simulink model "run_sim_paper_scenario"  (R2020a)
settings: Solver=ode4  StartTime=0.0  StopTime=30.0  FixedStep=0.01  RelTol=1e-3
values from neighbouring files (symbols this model uses):
  alfa_theta = 20    [init_sim_paper_scenario.m]
  alfa_theta_obs = 100    [init_sim_paper_scenario.m]
  beta1 = 1.2    [init_sim_paper_scenario.m]
  beta2 = 0.8    [init_sim_paper_scenario.m]
  beta_Phi_1 = pp0 * cal_frac_squ( 3, p_p0_plus_1, q_p0_plus_1 )                          * cal_frac_squ( eps_s_bar / pi, p_p0_min_2, q_p0_min_2 )                          / ( 2 * ( 2 * pp0 - 1 ) * tanh( gamma0 * ( eps_s_bar / pi ) / 2 ) )                          - ( cal_frac_squ( 3, p_p0_plus_1, q_p0_plus_1 ) * gamma0 / ( 4 * ( 2 * pp0 -1 ) ) )                          * cal_frac_squ( eps_s_bar / pi, p_p0_min_ ...(+136 chars)    [init_sim_paper_scenario.m]
  beta_Phi_2 = ( 1 - pp0 ) * cal_frac_squ( 3, p_p0_plus_1, q_p0_plus_1 )                          / ( 2 * ( 1 - 2 * pp0 ) * cal_frac_squ( eps_s_bar / pi, p_p0_0, q_p0_0 ) * tanh( gamma0 * ( eps_s_bar / pi ) / 2 ) )                          - ( cal_frac_squ( 3, p_p0_plus_1, q_p0_plus_1 ) * gamma0 / ( 4 * ( 1 - 2 * pp0 ) ) )                          * cal_frac_squ( eps_s_bar / pi, p_1_min_p0, q_1_min_p0 )          ...(+112 chars)    [init_sim_paper_scenario.m]
  c1_diff_sigma_bar_v = diag([25; 30; 20])    [init_sim_paper_scenario.m]
  c1_diff_sigma_bar_w = diag([12; 12; 12])    [init_sim_paper_scenario.m]
  c1_diff_ui = diag([25; 30; 20])    [init_sim_paper_scenario.m]
  c1v = diag([5.8; 6.5; 6.5])    [init_sim_paper_scenario.m]
  c2_diff_sigma_bar_v = diag([50; 50; 10])    [init_sim_paper_scenario.m]
  c2_diff_sigma_bar_w = diag([12; 12; 12])    [init_sim_paper_scenario.m]
  c2_diff_ui = diag([50; 50; 10])    [init_sim_paper_scenario.m]
  c2v = diag([5.8; 6.5; 6.5])    [init_sim_paper_scenario.m]
  c3_diff_sigma_bar_v = diag([15; 15; 10])    [init_sim_paper_scenario.m]
  c3_diff_sigma_bar_w = diag([15; 15; 15])    [init_sim_paper_scenario.m]
  c3_diff_ui = diag([15; 15; 10])    [init_sim_paper_scenario.m]
  c3v = diag([4.8; 6.4; 6.0])    [init_sim_paper_scenario.m]
  c_w_1 = diag( [20; 15; 15] )    [init_sim_paper_scenario.m]
  c_w_2 = diag( [20; 15; 15] )    [init_sim_paper_scenario.m]
  c_w_3 = diag( [2; 2; 2] )    [init_sim_paper_scenario.m]
  cS0 = diag( [4.5; 4.5; 4.5] )    [init_sim_paper_scenario.m]
  delta_p_i_0 = zeros(3, NF)    [init_sim_paper_scenario.m]
  delta_v_i_0 = zeros(3, NF)    [init_sim_paper_scenario.m]
  dp_aa_t = 0.2 * ones(3, 5) + ( 1.0 - 0.2 ) * rand(3, 5)    [init_sim_paper_scenario.m]
  dp_ff_t = [ 0.4 * ones(1, 5) + ( 1.0 - 0.4 ) * rand(1, 5);                      0.4 * ones(1, 5) + ( 1.0 - 0.4 ) * rand(1, 5);                      0.2 * ones(1, 5) + ( 0.6 - 0.2 ) * rand(1, 5) ]    [init_sim_paper_scenario.m]
  dp_phi_t = ( - pi / 2 ) * ones(3, 5) + ( pi / 2 - ( - pi / 2 ) ) * rand(3, 5)    [init_sim_paper_scenario.m]
  dw_aa_t = 0.2 * ones(3, 5) + ( 1.0 - 0.2 ) * rand(3, 5)    [init_sim_paper_scenario.m]
  dw_ff_t = [ 0.4 * ones(1, 5) + ( 1.0 - 0.4 ) * rand(1, 5);                      0.4 * ones(1, 5) + ( 1.0 - 0.4 ) * rand(1, 5);                      0.2 * ones(1, 5) + ( 0.6 - 0.2 ) * rand(1, 5) ]    [init_sim_paper_scenario.m]
  dw_phi_t = ( - pi / 2 ) * ones(3, 5) + ( pi / 2 - ( - pi / 2 ) ) * rand(3, 5)    [init_sim_paper_scenario.m]
  dwci_init = zeros(3,5)    [init_sim_paper_scenario.m]
  eps_s_bar_div_pi = eps_s_bar / pi    (= 0.03)    [init_sim_paper_scenario.m]
  etai_0 = zeros(3,5)    [init_sim_paper_scenario.m]
  gamma0 = 20    [init_sim_paper_scenario.m]
  h1w = diag([20.0; 20.0; 20.0])    [init_sim_paper_scenario.m]
  h2w = diag([30.0; 35.0; 35.0])    [init_sim_paper_scenario.m]
  h3w = diag([30.0; 25.0; 30.0])    [init_sim_paper_scenario.m]
  Ji = zeros(3,3,NF)    [init_sim_paper_scenario.m]
  k_J_0 = diag( [1; 1; 1] )    [init_sim_paper_scenario.m]
  kai_1_t = 0.02    [init_sim_paper_scenario.m]
  kai_3_t = 0.1    [init_sim_paper_scenario.m]
  kai_chi_1 = diag([6; 6; 6])    [init_sim_paper_scenario.m]
  kai_chi_2 = diag([6; 6; 6])    [init_sim_paper_scenario.m]
  kai_u_1 = diag([8; 8; 8])    [init_sim_paper_scenario.m]
  kai_u_2 = diag([8; 8; 8])    [init_sim_paper_scenario.m]
  ksii_0 = zeros(3,5)    [init_sim_paper_scenario.m]
  l1v = diag([20; 20; 20])    [init_sim_paper_scenario.m]
  l2v = diag([30; 30; 30])    [init_sim_paper_scenario.m]
  Lamd_diff_sigma_bar_v = 0.5    [init_sim_paper_scenario.m]
  Lamd_diff_sigma_bar_w = 0.8    [init_sim_paper_scenario.m]
  Lamd_diff_ui = 0.8    [init_sim_paper_scenario.m]
  mass_i = zeros(1,NF)    [init_sim_paper_scenario.m]
  Mii = diag([1;0;0;0;1])    [init_sim_paper_scenario.m]
  mu_c_theta = 100    [init_sim_paper_scenario.m]
  mu_d_w = 100    [init_sim_paper_scenario.m]
  pos0 = zeros(3, 1)    [init_sim_paper_scenario.m]
  pp0 = 8 / 11    (= 0.727272727273)    [init_sim_paper_scenario.m]    (also in plot_sim_paper_scenario.m = plot3( ksi0(1, kkt), ksi0(2, kkt), ksi0(3, kkt),            )
  PZ0 = P0(3)    [init_sim_paper_scenario.m]
  PZ1 = 10    [init_sim_paper_scenario.m]
  Qci_init = repmat([1;0;0;0],1,NF)    [init_sim_paper_scenario.m]
  R0 = 4    [init_sim_paper_scenario.m]
  R1 = 8    [init_sim_paper_scenario.m]
  Rci_init = zeros(3,3,NF)    [init_sim_paper_scenario.m]
  Ri_init = zeros(3,3,NF)    [init_sim_paper_scenario.m]
  Rx2 = 10    [init_sim_paper_scenario.m]
  Ry2 = 6    [init_sim_paper_scenario.m]
  Rz2 = 4    [init_sim_paper_scenario.m]
  T0 = 0    [init_sim_paper_scenario.m]
  T1 = tseq1    (= 10)    [init_sim_paper_scenario.m]
  T12 = tseq1 + tseq12    (= 20)    [init_sim_paper_scenario.m]
  T2 = tseq1 + tseq12 + tseq2    (= 30)    [init_sim_paper_scenario.m]
  theta0 = ( 2 / 5 ) * pi    (= 1.25663706144)    [init_sim_paper_scenario.m]
  thr_p_plus_1 = cal_frac_squ( 3, p_p0_plus_1, q_p0_plus_1 )    [init_sim_paper_scenario.m]
  ui_init = zeros(3,NF)    [init_sim_paper_scenario.m]
  vel0 = zeros(3, 1)    [init_sim_paper_scenario.m]
  wci_init = zeros(3,5)    [init_sim_paper_scenario.m]
  Wij = [0,0,1,0,0;              0,0,1,1,0;              1,0,0,0,1;              0,1,1,0,0;              0,0,1,0,0]    [init_sim_paper_scenario.m]
  X1 = 8    [init_sim_paper_scenario.m]
  X2 = 2    [init_sim_paper_scenario.m]
  X3 = 3    [init_sim_paper_scenario.m]
  Y1 = 10    [init_sim_paper_scenario.m]
  Y2 = 2    [init_sim_paper_scenario.m]
  Y3 = 4    [init_sim_paper_scenario.m]
  Z1 = 4    [init_sim_paper_scenario.m]
  Z2 = -6    [init_sim_paper_scenario.m]
  Z3 = 2    [init_sim_paper_scenario.m]
  zeta_diff_sigma_bar_v = 0.08    [init_sim_paper_scenario.m]
  zeta_diff_sigma_bar_w = 0.3    [init_sim_paper_scenario.m]
  zeta_diff_ui = 0.05    [init_sim_paper_scenario.m]
undefined symbols (not defined in the file or in its folder): cal_frac_squ, p_2_p0, p_alfav1, p_alfav2, p_alfaw1, p_alfaw2, p_beta1, p_beta2, p_beta_w_1, p_beta_w_2, p_dbeta1, p_dbeta2, p_gamma1_pos, p_gamma1_vel, p_gamma2_pos, p_gamma2_vel, p_p0_min_1, p_p0_plus_1, q_2_p0, q_alfav1, q_alfav2, q_alfaw1, q_alfaw2, q_beta1, q_beta2, q_beta_w_1, q_beta_w_2, q_dbeta1, q_dbeta2, q_gamma1_pos, q_gamma1_vel, q_gamma2_pos, q_gamma2_vel, q_p0_min_1, q_p0_plus_1, Qei_init, Qi_init, Rei_init, V_Phi_Rei_init, wei_init, wi_init
(part 8 of 10)

== matlab function run_sim_paper_scenario/cal abs 72 ==
  data: x input; y output
function y = fcn(x)
y = abs(x(:));

== matlab function run_sim_paper_scenario/cal abs 73 ==
  data: x input; y output
function y = fcn(x)
y = abs(x(:));

== matlab function run_sim_paper_scenario/cal abs 74 ==
  data: x input; y output
function y = fcn(x)
y = abs(x(:));

== matlab function run_sim_paper_scenario/cal abs 75 ==
  data: x input; y output
function y = fcn(x)
y = abs(x(:));

== matlab function run_sim_paper_scenario/cal abs 76 ==
  data: x input; y output
function y = fcn(x)
y = abs(x(:));

== matlab function run_sim_paper_scenario/cal abs 77 ==
  data: x input; y output
function y = fcn(x)
y = abs(x(:));

== matlab function run_sim_paper_scenario/cal abs 78 ==
  data: x input; y output
function y = fcn(x)
y = abs(x(:));

== matlab function run_sim_paper_scenario/cal abs 79 ==
  data: x input; y output
function y = fcn(x)
y = abs(x(:));

== matlab function run_sim_paper_scenario/cal abs 80 ==
  data: x input; y output
function y = fcn(x)
y = abs(x(:));

== matlab function run_sim_paper_scenario/cal abs 81 ==
  data: x input; y output
function y = fcn(x)
y = abs(x(:));

== matlab function run_sim_paper_scenario/trans to column6 ==
  data: x input; y output
function y = fcn(x)
y = x(:);

== matlab function run_sim_paper_scenario/cal abs 82 ==
  data: x input; y output
function y = fcn(x)
y = abs(x(:));

== matlab function run_sim_paper_scenario/cal abs 83 ==
  data: x input; y output
function y = fcn(x)
y = abs(x(:));

== matlab function run_sim_paper_scenario/cal abs 84 ==
  data: x input; y output
function y = fcn(x)
y = abs(x(:));

== matlab function run_sim_paper_scenario/cal abs 85 ==
  data: x input; y output
function y = fcn(x)
y = abs(x(:));

== matlab function run_sim_paper_scenario/cal abs 86 ==
  data: x input; y output
function y = fcn(x)
y = abs(x(:));

== matlab function run_sim_paper_scenario/cal abs 87 ==
  data: x input; y output
function y = fcn(x)
y = abs(x(:));

== matlab function run_sim_paper_scenario/cal abs 88 ==
  data: x input; y output
function y = fcn(x)
y = abs(x(:));

== matlab function run_sim_paper_scenario/cal abs 89 ==
  data: x input; y output
function y = fcn(x)
y = abs(x(:));

== matlab function run_sim_paper_scenario/cal abs 90 ==
  data: x input; y output
function y = fcn(x)
y = abs(x(:));

== matlab function run_sim_paper_scenario/cal abs 91 ==
  data: x input; y output
function y = fcn(x)
y = abs(x(:));

== matlab function run_sim_paper_scenario/trans to column7 ==
  data: x input; y output
function y = fcn(x)
y = x(:);

== matlab function run_sim_paper_scenario/cal abs 92 ==
  data: x input; y output
function y = fcn(x)
y = abs(x(:));

== matlab function run_sim_paper_scenario/cal abs 93 ==
  data: x input; y output
function y = fcn(x)
y = abs(x(:));

== matlab function run_sim_paper_scenario/cal abs 94 ==
  data: x input; y output
function y = fcn(x)
y = abs(x(:));

== matlab function run_sim_paper_scenario/cal abs 95 ==
  data: x input; y output
function y = fcn(x)
y = abs(x(:));

== matlab function run_sim_paper_scenario/cal combine sigma_bar_w_tilt ==
  data: sigma_bar_w_vec input; sigma_bar_w_hat_vec input; sigma_bar_w_tilt_vec output
function sigma_bar_w_tilt_vec = fcn(sigma_bar_w_vec, sigma_bar_w_hat_vec)
%%%% observation error of virtual angular velocity control variable
sigma_bar_w_tilt_vec = zeros(3,5);
for iiuav = 1:5
    sigma_bar_w_tilt_vec(:,iiuav) = sigma_bar_w_vec(:,iiuav) - sigma_bar_w_hat_vec(:,iiuav);
end

== matlab function run_sim_paper_scenario/cal d_sigma_w agent 1 ==
  data: h3w input; d_sigma_w_1 output; Ji input; wi_vec input; taui_vec input; sigma_w_bar_vec input
function d_sigma_w_1 = fcn(h3w, Ji, wi_vec, taui_vec, sigma_w_bar_vec)
%%%% auxiliary angular velocity derivative
iiuav = 1;
d_sigma_w_1 = inv(Ji(:,:,iiuav)) * ( -cal_askew_mat(wi_vec(:,iiuav)) * Ji(:,:,iiuav) * wi_vec(:,iiuav) ...
                            + taui_vec(:,iiuav) + h3w * sigma_w_bar_vec(:,iiuav) );

== matlab function run_sim_paper_scenario/cal d_sigma_w agent 2 ==
  data: h3w input; d_sigma_w_2 output; Ji input; wi_vec input; taui_vec input; sigma_w_bar_vec input
function d_sigma_w_2 = fcn(h3w, Ji, wi_vec, taui_vec, sigma_w_bar_vec)
%%%% auxiliary angular velocity derivative
iiuav = 2;
d_sigma_w_2 = inv(Ji(:,:,iiuav)) * ( -cal_askew_mat(wi_vec(:,iiuav)) * Ji(:,:,iiuav) * wi_vec(:,iiuav) ...
                            + taui_vec(:,iiuav) + h3w * sigma_w_bar_vec(:,iiuav) );

== matlab function run_sim_paper_scenario/cal d_sigma_w agent 3 ==
  data: h3w input; d_sigma_w_3 output; Ji input; wi_vec input; taui_vec input; sigma_w_bar_vec input
function d_sigma_w_3 = fcn(h3w, Ji, wi_vec, taui_vec, sigma_w_bar_vec)
%%%% auxiliary angular velocity derivative
iiuav = 3;
d_sigma_w_3 = inv(Ji(:,:,iiuav)) * ( -cal_askew_mat(wi_vec(:,iiuav)) * Ji(:,:,iiuav) * wi_vec(:,iiuav) ...
                            + taui_vec(:,iiuav) + h3w * sigma_w_bar_vec(:,iiuav) );

== matlab function run_sim_paper_scenario/uav translational dynamics agent 1 ==
  data: dvi output; Ri input; ui input; dp input
function dvi = fcn(Ri, ui, dp)
%%%% update translational velocity dynamics
iiuav = 1;
g0 = 9.80663;
e3 = [0;0;1];
dvi = -g0 * e3 + norm(ui(:,iiuav),2) * Ri(:,:,iiuav) * e3 + dp(:,iiuav);

== matlab function run_sim_paper_scenario/cal d_sigma_w agent 4 ==
  data: h3w input; d_sigma_w_4 output; Ji input; wi_vec input; taui_vec input; sigma_w_bar_vec input
function d_sigma_w_4 = fcn(h3w, Ji, wi_vec, taui_vec, sigma_w_bar_vec)
%%%% auxiliary angular velocity derivative
iiuav = 4;
d_sigma_w_4 = inv(Ji(:,:,iiuav)) * ( -cal_askew_mat(wi_vec(:,iiuav)) * Ji(:,:,iiuav) * wi_vec(:,iiuav) ...
                            + taui_vec(:,iiuav) + h3w * sigma_w_bar_vec(:,iiuav) );

== matlab function run_sim_paper_scenario/cal d_sigma_w agent 5 ==
  data: h3w input; d_sigma_w_5 output; Ji input; wi_vec input; taui_vec input; sigma_w_bar_vec input
function d_sigma_w_5 = fcn(h3w, Ji, wi_vec, taui_vec, sigma_w_bar_vec)
%%%% auxiliary angular velocity derivative
iiuav = 5;
d_sigma_w_5 = inv(Ji(:,:,iiuav)) * ( -cal_askew_mat(wi_vec(:,iiuav)) * Ji(:,:,iiuav) * wi_vec(:,iiuav) ...
                            + taui_vec(:,iiuav) + h3w * sigma_w_bar_vec(:,iiuav) );

== matlab function run_sim_paper_scenario/cal duihat d2uihat by high-order differentiator node 1 ==
  data: c1 input; d_ui_hat output; d_dui_hat output; d_d2ui_hat output; c2 input; c3 input; chi_t input; ui_sig_1 input; ui_sig_2 input; ui_sig_3 input; ui_sig_4 input; ui_sig_5 input; ui_sig_6 input; dui_hat input; d2ui_hat input
function [d_ui_hat, d_dui_hat, d_d2ui_hat] = fcn(c1, c2, c3, chi_t, ui_sig_1, ui_sig_2, ui_sig_3, ...
                                                                                        ui_sig_4, ui_sig_5, ui_sig_6, dui_hat, d2ui_hat)
%%%% high-order sliding mode differentiator
d_d2ui_hat = -chi_t .* c1 * ui_sig_1(:) - (1 - chi_t) .* c1 * ui_sig_2(:);
d_dui_hat = -chi_t .* c2 * ui_sig_3(:) - (1 - chi_t) .* c2 * ui_sig_4(:) + d2ui_hat(:);
d_ui_hat = -chi_t .* c3 * ui_sig_5(:) - (1 - chi_t) .* c3 * ui_sig_6(:) + dui_hat(:);

== matlab function run_sim_paper_scenario/cal duihat d2uihat by high-order differentiator node 2 ==
  data: c1 input; d_ui_hat output; d_dui_hat output; d_d2ui_hat output; c2 input; c3 input; chi_t input; ui_sig_1 input; ui_sig_2 input; ui_sig_3 input; ui_sig_4 input; ui_sig_5 input; ui_sig_6 input; dui_hat input; d2ui_hat input
function [d_ui_hat, d_dui_hat, d_d2ui_hat] = fcn(c1, c2, c3, chi_t, ui_sig_1, ui_sig_2, ui_sig_3, ...
                                                                                        ui_sig_4, ui_sig_5, ui_sig_6, dui_hat, d2ui_hat)
%%%% high-order sliding mode differentiator
d_d2ui_hat = -chi_t .* c1 * ui_sig_1(:) - (1 - chi_t) .* c1 * ui_sig_2(:);
d_dui_hat = -chi_t .* c2 * ui_sig_3(:) - (1 - chi_t) .* c2 * ui_sig_4(:) + d2ui_hat(:);
d_ui_hat = -chi_t .* c3 * ui_sig_5(:) - (1 - chi_t) .* c3 * ui_sig_6(:) + dui_hat(:);

== matlab function run_sim_paper_scenario/cal duihat d2uihat by high-order differentiator node 3 ==
  data: c1 input; d_ui_hat output; d_dui_hat output; d_d2ui_hat output; c2 input; c3 input; chi_t input; ui_sig_1 input; ui_sig_2 input; ui_sig_3 input; ui_sig_4 input; ui_sig_5 input; ui_sig_6 input; dui_hat input; d2ui_hat input
function [d_ui_hat, d_dui_hat, d_d2ui_hat] = fcn(c1, c2, c3, chi_t, ui_sig_1, ui_sig_2, ui_sig_3, ...
                                                                                        ui_sig_4, ui_sig_5, ui_sig_6, dui_hat, d2ui_hat)
%%%% high-order sliding mode differentiator
d_d2ui_hat = -chi_t .* c1 * ui_sig_1(:) - (1 - chi_t) .* c1 * ui_sig_2(:);
d_dui_hat = -chi_t .* c2 * ui_sig_3(:) - (1 - chi_t) .* c2 * ui_sig_4(:) + d2ui_hat(:);
d_ui_hat = -chi_t .* c3 * ui_sig_5(:) - (1 - chi_t) .* c3 * ui_sig_6(:) + dui_hat(:);

== matlab function run_sim_paper_scenario/cal duihat d2uihat by high-order differentiator node 4 ==
  data: c1 input; d_ui_hat output; d_dui_hat output; d_d2ui_hat output; c2 input; c3 input; chi_t input; ui_sig_1 input; ui_sig_2 input; ui_sig_3 input; ui_sig_4 input; ui_sig_5 input; ui_sig_6 input; dui_hat input; d2ui_hat input
function [d_ui_hat, d_dui_hat, d_d2ui_hat] = fcn(c1, c2, c3, chi_t, ui_sig_1, ui_sig_2, ui_sig_3, ...
                                                                                        ui_sig_4, ui_sig_5, ui_sig_6, dui_hat, d2ui_hat)
%%%% high-order sliding mode differentiator
d_d2ui_hat = -chi_t .* c1 * ui_sig_1(:) - (1 - chi_t) .* c1 * ui_sig_2(:);
d_dui_hat = -chi_t .* c2 * ui_sig_3(:) - (1 - chi_t) .* c2 * ui_sig_4(:) + d2ui_hat(:);
d_ui_hat = -chi_t .* c3 * ui_sig_5(:) - (1 - chi_t) .* c3 * ui_sig_6(:) + dui_hat(:);

== matlab function run_sim_paper_scenario/uav translational dynamics agent 2 ==
  data: dvi output; Ri input; ui input; dp input
function dvi = fcn(Ri, ui, dp)
%%%% update translational velocity dynamics
iiuav = 2;
g0 = 9.80663;
e3 = [0;0;1];
dvi = -g0 * e3 + norm(ui(:,iiuav),2) * Ri(:,:,iiuav) * e3 + dp(:,iiuav);

== matlab function run_sim_paper_scenario/cal duihat d2uihat by high-order differentiator node 5 ==
  data: c1 input; d_ui_hat output; d_dui_hat output; d_d2ui_hat output; c2 input; c3 input; chi_t input; ui_sig_1 input; ui_sig_2 input; ui_sig_3 input; ui_sig_4 input; ui_sig_5 input; ui_sig_6 input; dui_hat input; d2ui_hat input
function [d_ui_hat, d_dui_hat, d_d2ui_hat] = fcn(c1, c2, c3, chi_t, ui_sig_1, ui_sig_2, ui_sig_3, ...
                                                                                        ui_sig_4, ui_sig_5, ui_sig_6, dui_hat, d2ui_hat)
%%%% high-order sliding mode differentiator
d_d2ui_hat = -chi_t .* c1 * ui_sig_1(:) - (1 - chi_t) .* c1 * ui_sig_2(:);
d_dui_hat = -chi_t .* c2 * ui_sig_3(:) - (1 - chi_t) .* c2 * ui_sig_4(:) + d2ui_hat(:);
d_ui_hat = -chi_t .* c3 * ui_sig_5(:) - (1 - chi_t) .* c3 * ui_sig_6(:) + dui_hat(:);

== matlab function run_sim_paper_scenario/cal differentiator d_sigma_bar_w_hat agent 1/cal differentiator ==
  data: c1 input; d_sigma_bar_v_hat output; d_dsigma_bar_v_hat output; d_d2sigma_bar_v_hat output; c2 input; c3 input; chi_t input; sigma_bar_v_sig_1 input; sigma_bar_v_sig_2 input; sigma_bar_v_sig_3 input; sigma_bar_v_sig_4 input; sigma_bar_v_sig_5 input; sigma_bar_v_sig_6 input; d_sigma_bar_v_hat input; d2_sigma_bar_v_hat input
function [d_sigma_bar_v_hat, d_dsigma_bar_v_hat, d_d2sigma_bar_v_hat] = fcn(c1, c2, c3, chi_t, sigma_bar_v_sig_1, sigma_bar_v_sig_2, sigma_bar_v_sig_3, ...
                                                                                                                                                sigma_bar_v_sig_4, sigma_bar_v_sig_5, sigma_bar_v_sig_6, d_sigma_bar_v_hat, d2_sigma_bar_v_hat)
d_d2sigma_bar_v_hat = -chi_t .* c1 * sigma_bar_v_sig_1(:) - (1 - chi_t) .* c1 * sigma_bar_v_sig_2(:);
d_dsigma_bar_v_hat = -chi_t .* c2 * sigma_bar_v_sig_3(:) - (1 - chi_t) .* c2 * sigma_bar_v_sig_4(:) + d2_sigma_bar_v_hat(:);
d_sigma_bar_v_hat = -chi_t .* c3 * sigma_bar_v_sig_5(:) - (1 - chi_t) .* c3 * sigma_bar_v_sig_6(:) + d_sigma_bar_v_hat(:);

== matlab function run_sim_paper_scenario/cal differentiator d_sigma_bar_w_hat agent 1/cal sig ==
  data: x input; z output; y input
function z = fcn(x, y)
z = x(:) .* sign(y(:));

== matlab function run_sim_paper_scenario/cal differentiator d_sigma_bar_w_hat agent 1/cal sig1 ==
  data: x input; z output; y input
function z = fcn(x, y)
z = x(:) .* sign(y(:));

== matlab function run_sim_paper_scenario/cal differentiator d_sigma_bar_w_hat agent 1/cal sig2 ==
  data: x input; z output; y input
function z = fcn(x, y)
z = x(:) .* sign(y(:));

== matlab function run_sim_paper_scenario/cal differentiator d_sigma_bar_w_hat agent 1/cal sig3 ==
  data: x input; z output; y input
function z = fcn(x, y)
z = x(:) .* sign(y(:));

== matlab function run_sim_paper_scenario/cal differentiator d_sigma_bar_w_hat agent 1/cal sig4 ==
  data: x input; z output; y input
function z = fcn(x, y)
z = x(:) .* sign(y(:));

== matlab function run_sim_paper_scenario/uav translational dynamics agent 3 ==
  data: dvi output; Ri input; ui input; dp input
function dvi = fcn(Ri, ui, dp)
%%%% update translational velocity dynamics
iiuav = 3;
g0 = 9.80663;
e3 = [0;0;1];
dvi = -g0 * e3 + norm(ui(:,iiuav),2) * Ri(:,:,iiuav) * e3 + dp(:,iiuav);

== matlab function run_sim_paper_scenario/cal differentiator d_sigma_bar_w_hat agent 1/cal sig5 ==
  data: x input; z output; y input
function z = fcn(x, y)
z = x(:) .* sign(y(:));

== matlab function run_sim_paper_scenario/cal differentiator d_sigma_bar_w_hat agent 1/choose sigma_bar_w ==
  data: x input; y output
function y = fcn(x)
iiuav = 1;
y = x(:,iiuav);

== matlab function run_sim_paper_scenario/cal differentiator d_sigma_bar_w_hat agent 1/trans to column20 ==
  data: x input; y output
function y = fcn(x)
y = x(:);

== matlab function run_sim_paper_scenario/cal differentiator d_sigma_bar_w_hat agent 1/trans to column21 ==
  data: x input; y output
function y = fcn(x)
y = x(:);

== matlab function run_sim_paper_scenario/cal differentiator d_sigma_bar_w_hat agent 1/trans to column22 ==
  data: x input; y output
function y = fcn(x)
y = x(:);

== matlab function run_sim_paper_scenario/cal differentiator d_sigma_bar_w_hat agent 1/trans to column23 ==
  data: x input; y output
function y = fcn(x)
y = x(:);

== matlab function run_sim_paper_scenario/cal differentiator d_sigma_bar_w_hat agent 1/trans to column24 ==
  data: x input; y output
function y = fcn(x)
y = x(:);

== matlab function run_sim_paper_scenario/cal differentiator d_sigma_bar_w_hat agent 1/trans to column25 ==
  data: x input; y output
function y = fcn(x)
y = x(:);

== matlab function run_sim_paper_scenario/cal differentiator d_sigma_bar_w_hat agent 2/cal differentiator ==
  data: c1 input; d_sigma_bar_v_hat output; d_dsigma_bar_v_hat output; d_d2sigma_bar_v_hat output; c2 input; c3 input; chi_t input; sigma_bar_v_sig_1 input; sigma_bar_v_sig_2 input; sigma_bar_v_sig_3 input; sigma_bar_v_sig_4 input; sigma_bar_v_sig_5 input; sigma_bar_v_sig_6 input; d_sigma_bar_v_hat input; d2_sigma_bar_v_hat input
function [d_sigma_bar_v_hat, d_dsigma_bar_v_hat, d_d2sigma_bar_v_hat] = fcn(c1, c2, c3, chi_t, sigma_bar_v_sig_1, sigma_bar_v_sig_2, sigma_bar_v_sig_3, ...
                                                                                                                                                sigma_bar_v_sig_4, sigma_bar_v_sig_5, sigma_bar_v_sig_6, d_sigma_bar_v_hat, d2_sigma_bar_v_hat)
d_d2sigma_bar_v_hat = -chi_t .* c1 * sigma_bar_v_sig_1(:) - (1 - chi_t) .* c1 * sigma_bar_v_sig_2(:);
d_dsigma_bar_v_hat = -chi_t .* c2 * sigma_bar_v_sig_3(:) - (1 - chi_t) .* c2 * sigma_bar_v_sig_4(:) + d2_sigma_bar_v_hat(:);
d_sigma_bar_v_hat = -chi_t .* c3 * sigma_bar_v_sig_5(:) - (1 - chi_t) .* c3 * sigma_bar_v_sig_6(:) + d_sigma_bar_v_hat(:);

== matlab function run_sim_paper_scenario/cal differentiator d_sigma_bar_w_hat agent 2/cal sig ==
  data: x input; z output; y input
function z = fcn(x, y)
z = x(:) .* sign(y(:));

== matlab function run_sim_paper_scenario/uav translational dynamics agent 4 ==
  data: dvi output; Ri input; ui input; dp input
function dvi = fcn(Ri, ui, dp)
%%%% update translational velocity dynamics
iiuav = 4;
g0 = 9.80663;
e3 = [0;0;1];
dvi = -g0 * e3 + norm(ui(:,iiuav),2) * Ri(:,:,iiuav) * e3 + dp(:,iiuav);

== matlab function run_sim_paper_scenario/cal differentiator d_sigma_bar_w_hat agent 2/cal sig1 ==
  data: x input; z output; y input
function z = fcn(x, y)
z = x(:) .* sign(y(:));

== matlab function run_sim_paper_scenario/cal differentiator d_sigma_bar_w_hat agent 2/cal sig2 ==
  data: x input; z output; y input
function z = fcn(x, y)
z = x(:) .* sign(y(:));

== matlab function run_sim_paper_scenario/cal differentiator d_sigma_bar_w_hat agent 2/cal sig3 ==
  data: x input; z output; y input
function z = fcn(x, y)
z = x(:) .* sign(y(:));

== matlab function run_sim_paper_scenario/cal differentiator d_sigma_bar_w_hat agent 2/cal sig4 ==
  data: x input; z output; y input
function z = fcn(x, y)
z = x(:) .* sign(y(:));

== matlab function run_sim_paper_scenario/cal differentiator d_sigma_bar_w_hat agent 2/cal sig5 ==
  data: x input; z output; y input
function z = fcn(x, y)
z = x(:) .* sign(y(:));

== matlab function run_sim_paper_scenario/cal differentiator d_sigma_bar_w_hat agent 2/choose sigma_bar_w ==
  data: x input; y output
function y = fcn(x)
iiuav = 2;
y = x(:,iiuav);

== matlab function run_sim_paper_scenario/cal differentiator d_sigma_bar_w_hat agent 2/trans to column20 ==
  data: x input; y output
function y = fcn(x)
y = x(:);

== matlab function run_sim_paper_scenario/cal differentiator d_sigma_bar_w_hat agent 2/trans to column21 ==
  data: x input; y output
function y = fcn(x)
y = x(:);

== matlab function run_sim_paper_scenario/cal differentiator d_sigma_bar_w_hat agent 2/trans to column22 ==
  data: x input; y output
function y = fcn(x)
y = x(:);

== matlab function run_sim_paper_scenario/cal differentiator d_sigma_bar_w_hat agent 2/trans to column23 ==
  data: x input; y output
function y = fcn(x)
y = x(:);

== matlab function run_sim_paper_scenario/cal differentiator d_sigma_bar_w_hat agent 2/trans to column24 ==
  data: x input; y output
function y = fcn(x)
y = x(:);

== matlab function run_sim_paper_scenario/cal differentiator d_sigma_bar_w_hat agent 2/trans to column25 ==
  data: x input; y output
function y = fcn(x)
y = x(:);

== matlab function run_sim_paper_scenario/uav translational dynamics agent 5 ==
  data: dvi output; Ri input; ui input; dp input
function dvi = fcn(Ri, ui, dp)
%%%% update translational velocity dynamics
iiuav = 5;
g0 = 9.80663;
e3 = [0;0;1];
dvi = -g0 * e3 + norm(ui(:,iiuav),2) * Ri(:,:,iiuav) * e3 + dp(:,iiuav);

== matlab function run_sim_paper_scenario/cal differentiator d_sigma_bar_w_hat agent 3/cal differentiator ==
  data: c1 input; d_sigma_bar_v_hat output; d_dsigma_bar_v_hat output; d_d2sigma_bar_v_hat output; c2 input; c3 input; chi_t input; sigma_bar_v_sig_1 input; sigma_bar_v_sig_2 input; sigma_bar_v_sig_3 input; sigma_bar_v_sig_4 input; sigma_bar_v_sig_5 input; sigma_bar_v_sig_6 input; d_sigma_bar_v_hat input; d2_sigma_bar_v_hat input
function [d_sigma_bar_v_hat, d_dsigma_bar_v_hat, d_d2sigma_bar_v_hat] = fcn(c1, c2, c3, chi_t, sigma_bar_v_sig_1, sigma_bar_v_sig_2, sigma_bar_v_sig_3, ...
                                                                                                                                                sigma_bar_v_sig_4, sigma_bar_v_sig_5, sigma_bar_v_sig_6, d_sigma_bar_v_hat, d2_sigma_bar_v_hat)
d_d2sigma_bar_v_hat = -chi_t .* c1 * sigma_bar_v_sig_1(:) - (1 - chi_t) .* c1 * sigma_bar_v_sig_2(:);
d_dsigma_bar_v_hat = -chi_t .* c2 * sigma_bar_v_sig_3(:) - (1 - chi_t) .* c2 * sigma_bar_v_sig_4(:) + d2_sigma_bar_v_hat(:);
d_sigma_bar_v_hat = -chi_t .* c3 * sigma_bar_v_sig_5(:) - (1 - chi_t) .* c3 * sigma_bar_v_sig_6(:) + d_sigma_bar_v_hat(:);

== matlab function run_sim_paper_scenario/cal differentiator d_sigma_bar_w_hat agent 3/cal sig ==
  data: x input; z output; y input
function z = fcn(x, y)
z = x(:) .* sign(y(:));

== matlab function run_sim_paper_scenario/cal differentiator d_sigma_bar_w_hat agent 3/cal sig1 ==
  data: x input; z output; y input
function z = fcn(x, y)
z = x(:) .* sign(y(:));

== matlab function run_sim_paper_scenario/cal differentiator d_sigma_bar_w_hat agent 3/cal sig2 ==
  data: x input; z output; y input
function z = fcn(x, y)
z = x(:) .* sign(y(:));

== matlab function run_sim_paper_scenario/cal differentiator d_sigma_bar_w_hat agent 3/cal sig3 ==
  data: x input; z output; y input
function z = fcn(x, y)
z = x(:) .* sign(y(:));

== matlab function run_sim_paper_scenario/cal differentiator d_sigma_bar_w_hat agent 3/cal sig4 ==
  data: x input; z output; y input
function z = fcn(x, y)
z = x(:) .* sign(y(:));

== matlab function run_sim_paper_scenario/cal differentiator d_sigma_bar_w_hat agent 3/cal sig5 ==
  data: x input; z output; y input
function z = fcn(x, y)
z = x(:) .* sign(y(:));

== matlab function run_sim_paper_scenario/cal differentiator d_sigma_bar_w_hat agent 3/choose sigma_bar_w ==
  data: x input; y output
function y = fcn(x)
iiuav = 3;
y = x(:,iiuav);

== matlab function run_sim_paper_scenario/cal differentiator d_sigma_bar_w_hat agent 3/trans to column20 ==
  data: x input; y output
function y = fcn(x)
y = x(:);

== matlab function run_sim_paper_scenario/cal differentiator d_sigma_bar_w_hat agent 3/trans to column21 ==
  data: x input; y output
function y = fcn(x)
y = x(:);

== matlab function run_sim_paper_scenario/cal Ri ==
  data: Ri output; Rei input; Rci input
function Ri = fcn(Rei, Rci)
Ri = zeros(3,3,5);
for iiuav = 1:5
    Ri(:,:,iiuav) = Rci(:,:,iiuav) * Rei(:,:,iiuav);
end

end

== matlab function run_sim_paper_scenario/cal differentiator d_sigma_bar_w_hat agent 3/trans to column22 ==
  data: x input; y output
function y = fcn(x)
y = x(:);

== matlab function run_sim_paper_scenario/cal differentiator d_sigma_bar_w_hat agent 3/trans to column23 ==
  data: x input; y output
function y = fcn(x)
y = x(:);

== matlab function run_sim_paper_scenario/cal differentiator d_sigma_bar_w_hat agent 3/trans to column24 ==
  data: x input; y output
function y = fcn(x)
y = x(:);

== matlab function run_sim_paper_scenario/cal differentiator d_sigma_bar_w_hat agent 3/trans to column25 ==
  data: x input; y output
function y = fcn(x)
y = x(:);

== matlab function run_sim_paper_scenario/cal differentiator d_sigma_bar_w_hat agent 4/cal differentiator ==
  data: c1 input; d_sigma_bar_v_hat output; d_dsigma_bar_v_hat output; d_d2sigma_bar_v_hat output; c2 input; c3 input; chi_t input; sigma_bar_v_sig_1 input; sigma_bar_v_sig_2 input; sigma_bar_v_sig_3 input; sigma_bar_v_sig_4 input; sigma_bar_v_sig_5 input; sigma_bar_v_sig_6 input; d_sigma_bar_v_hat input; d2_sigma_bar_v_hat input
function [d_sigma_bar_v_hat, d_dsigma_bar_v_hat, d_d2sigma_bar_v_hat] = fcn(c1, c2, c3, chi_t, sigma_bar_v_sig_1, sigma_bar_v_sig_2, sigma_bar_v_sig_3, ...
                                                                                                                                                sigma_bar_v_sig_4, sigma_bar_v_sig_5, sigma_bar_v_sig_6, d_sigma_bar_v_hat, d2_sigma_bar_v_hat)
d_d2sigma_bar_v_hat = -chi_t .* c1 * sigma_bar_v_sig_1(:) - (1 - chi_t) .* c1 * sigma_bar_v_sig_2(:);
d_dsigma_bar_v_hat = -chi_t .* c2 * sigma_bar_v_sig_3(:) - (1 - chi_t) .* c2 * sigma_bar_v_sig_4(:) + d2_sigma_bar_v_hat(:);
d_sigma_bar_v_hat = -chi_t .* c3 * sigma_bar_v_sig_5(:) - (1 - chi_t) .* c3 * sigma_bar_v_sig_6(:) + d_sigma_bar_v_hat(:);

== matlab function run_sim_paper_scenario/cal differentiator d_sigma_bar_w_hat agent 4/cal sig ==
  data: x input; z output; y input
function z = fcn(x, y)
z = x(:) .* sign(y(:));

== matlab function run_sim_paper_scenario/cal differentiator d_sigma_bar_w_hat agent 4/cal sig1 ==
  data: x input; z output; y input
function z = fcn(x, y)
z = x(:) .* sign(y(:));

== matlab function run_sim_paper_scenario/cal differentiator d_sigma_bar_w_hat agent 4/cal sig2 ==
  data: x input; z output; y input
function z = fcn(x, y)
z = x(:) .* sign(y(:));

== matlab function run_sim_paper_scenario/cal differentiator d_sigma_bar_w_hat agent 4/cal sig3 ==
  data: x input; z output; y input
function z = fcn(x, y)
z = x(:) .* sign(y(:));

== matlab function run_sim_paper_scenario/follower tracking error agent 1 ==
  data: ksi_track_err_1 output; delta_ksi_vec input; delta_eta_vec input; ksi_i_vec input; eta_i_vec input; ksi0 input; eta_track_err_1 output; eta0 input
function [ksi_track_err_1, eta_track_err_1]  = fcn(delta_ksi_vec, delta_eta_vec, ksi_i_vec, eta_i_vec, ksi0, eta0)
%%%% translational state tracking error for followers
eta_track_err_1 = eta_i_vec(:,1) - delta_eta_vec(:,1) - eta0;
ksi_track_err_1 = ksi_i_vec(:,1) - delta_ksi_vec(:,1) - ksi0;

== matlab function run_sim_paper_scenario/cal differentiator d_sigma_bar_w_hat agent 4/cal sig4 ==
  data: x input; z output; y input
function z = fcn(x, y)
z = x(:) .* sign(y(:));

== matlab function run_sim_paper_scenario/cal differentiator d_sigma_bar_w_hat agent 4/cal sig5 ==
  data: x input; z output; y input
function z = fcn(x, y)
z = x(:) .* sign(y(:));

== matlab function run_sim_paper_scenario/cal differentiator d_sigma_bar_w_hat agent 4/choose sigma_bar_w ==
  data: x input; y output
function y = fcn(x)
iiuav = 4;
y = x(:,iiuav);

== matlab function run_sim_paper_scenario/cal differentiator d_sigma_bar_w_hat agent 4/trans to column20 ==
  data: x input; y output
function y = fcn(x)
y = x(:);

== matlab function run_sim_paper_scenario/cal differentiator d_sigma_bar_w_hat agent 4/trans to column21 ==
  data: x input; y output
function y = fcn(x)
y = x(:);

== matlab function run_sim_paper_scenario/cal differentiator d_sigma_bar_w_hat agent 4/trans to column22 ==
  data: x input; y output
function y = fcn(x)
y = x(:);

== matlab function run_sim_paper_scenario/cal differentiator d_sigma_bar_w_hat agent 4/trans to column23 ==
  data: x input; y output
function y = fcn(x)
y = x(:);

== matlab function run_sim_paper_scenario/cal differentiator d_sigma_bar_w_hat agent 4/trans to column24 ==
  data: x input; y output
function y = fcn(x)
y = x(:);

== matlab function run_sim_paper_scenario/cal differentiator d_sigma_bar_w_hat agent 4/trans to column25 ==
  data: x input; y output
function y = fcn(x)
y = x(:);

== matlab function run_sim_paper_scenario/cal differentiator d_sigma_bar_w_hat agent 5/cal differentiator ==
  data: c1 input; d_sigma_bar_v_hat output; d_dsigma_bar_v_hat output; d_d2sigma_bar_v_hat output; c2 input; c3 input; chi_t input; sigma_bar_v_sig_1 input; sigma_bar_v_sig_2 input; sigma_bar_v_sig_3 input; sigma_bar_v_sig_4 input; sigma_bar_v_sig_5 input; sigma_bar_v_sig_6 input; d_sigma_bar_v_hat input; d2_sigma_bar_v_hat input
function [d_sigma_bar_v_hat, d_dsigma_bar_v_hat, d_d2sigma_bar_v_hat] = fcn(c1, c2, c3, chi_t, sigma_bar_v_sig_1, sigma_bar_v_sig_2, sigma_bar_v_sig_3, ...
                                                                                                                                                sigma_bar_v_sig_4, sigma_bar_v_sig_5, sigma_bar_v_sig_6, d_sigma_bar_v_hat, d2_sigma_bar_v_hat)
d_d2sigma_bar_v_hat = -chi_t .* c1 * sigma_bar_v_sig_1(:) - (1 - chi_t) .* c1 * sigma_bar_v_sig_2(:);
d_dsigma_bar_v_hat = -chi_t .* c2 * sigma_bar_v_sig_3(:) - (1 - chi_t) .* c2 * sigma_bar_v_sig_4(:) + d2_sigma_bar_v_hat(:);
d_sigma_bar_v_hat = -chi_t .* c3 * sigma_bar_v_sig_5(:) - (1 - chi_t) .* c3 * sigma_bar_v_sig_6(:) + d_sigma_bar_v_hat(:);

== matlab function run_sim_paper_scenario/cal differentiator d_sigma_bar_w_hat agent 5/cal sig ==
  data: x input; z output; y input
function z = fcn(x, y)
z = x(:) .* sign(y(:));

== matlab function run_sim_paper_scenario/cal differentiator d_sigma_bar_w_hat agent 5/cal sig1 ==
  data: x input; z output; y input
function z = fcn(x, y)
z = x(:) .* sign(y(:));

== matlab function run_sim_paper_scenario/cal differentiator d_sigma_bar_w_hat agent 5/cal sig2 ==
  data: x input; z output; y input
function z = fcn(x, y)
z = x(:) .* sign(y(:));

== matlab function run_sim_paper_scenario/cal differentiator d_sigma_bar_w_hat agent 5/cal sig3 ==
  data: x input; z output; y input
function z = fcn(x, y)
z = x(:) .* sign(y(:));

== matlab function run_sim_paper_scenario/cal differentiator d_sigma_bar_w_hat agent 5/cal sig4 ==
  data: x input; z output; y input
function z = fcn(x, y)
z = x(:) .* sign(y(:));

== matlab function run_sim_paper_scenario/cal differentiator d_sigma_bar_w_hat agent 5/cal sig5 ==
  data: x input; z output; y input
function z = fcn(x, y)
z = x(:) .* sign(y(:));

== matlab function run_sim_paper_scenario/follower tracking error agent 2 ==
  data: ksi_track_err_2 output; delta_ksi_vec input; delta_eta_vec input; ksi_i_vec input; eta_i_vec input; ksi0 input; eta_track_err_2 output; eta0 input
function [ksi_track_err_2, eta_track_err_2]  = fcn(delta_ksi_vec, delta_eta_vec, ksi_i_vec, eta_i_vec, ksi0, eta0)
%%%% translational state tracking error for followers
eta_track_err_2 = eta_i_vec(:,2) - delta_eta_vec(:,2) - eta0;
ksi_track_err_2 = ksi_i_vec(:,2) - delta_ksi_vec(:,2) - ksi0;

== matlab function run_sim_paper_scenario/cal differentiator d_sigma_bar_w_hat agent 5/choose sigma_bar_w ==
  data: x input; y output
function y = fcn(x)
iiuav = 5;
y = x(:,iiuav);

== matlab function run_sim_paper_scenario/cal differentiator d_sigma_bar_w_hat agent 5/trans to column20 ==
  data: x input; y output
function y = fcn(x)
y = x(:);

== matlab function run_sim_paper_scenario/cal differentiator d_sigma_bar_w_hat agent 5/trans to column21 ==
  data: x input; y output
function y = fcn(x)
y = x(:);

== matlab function run_sim_paper_scenario/cal differentiator d_sigma_bar_w_hat agent 5/trans to column22 ==
  data: x input; y output
function y = fcn(x)
y = x(:);

== matlab function run_sim_paper_scenario/cal differentiator d_sigma_bar_w_hat agent 5/trans to column23 ==
  data: x input; y output
function y = fcn(x)
y = x(:);

== matlab function run_sim_paper_scenario/cal differentiator d_sigma_bar_w_hat agent 5/trans to column24 ==
  data: x input; y output
function y = fcn(x)
y = x(:);

== matlab function run_sim_paper_scenario/cal differentiator d_sigma_bar_w_hat agent 5/trans to column25 ==
  data: x input; y output
function y = fcn(x)
y = x(:);

== matlab function run_sim_paper_scenario/cal divide pi ==
  data: x input; y output
function y = fcn(x)
y = x ./ pi;

== matlab function run_sim_paper_scenario/cal dw_hat agent 1 ==
  data: h3w input; Ji input; d_sigma_bar_w_vec input; sigma_bar_w_hat_vec input; dw_hat_1 output
function dw_hat_1 = fcn(h3w, Ji, d_sigma_bar_w_vec, sigma_bar_w_hat_vec)
%%%% rotational disturbance observation
iiuav = 1;
dw_hat_1 = Ji(:,:,iiuav) * d_sigma_bar_w_vec(:,iiuav) + h3w * sigma_bar_w_hat_vec(:,iiuav);

== matlab function run_sim_paper_scenario/cal dw_hat agent 2 ==
  data: h3w input; Ji input; d_sigma_bar_w_vec input; sigma_bar_w_hat_vec input; dw_hat_2 output
function dw_hat_2 = fcn(h3w, Ji, d_sigma_bar_w_vec, sigma_bar_w_hat_vec)
%%%% rotational disturbance observation
iiuav = 2;
dw_hat_2 = Ji(:,:,iiuav) * d_sigma_bar_w_vec(:,iiuav) + h3w * sigma_bar_w_hat_vec(:,iiuav);

== matlab function run_sim_paper_scenario/cal dw_hat agent 3 ==
  data: h3w input; Ji input; d_sigma_bar_w_vec input; sigma_bar_w_hat_vec input; dw_hat_3 output
function dw_hat_3 = fcn(h3w, Ji, d_sigma_bar_w_vec, sigma_bar_w_hat_vec)
%%%% rotational disturbance observation
iiuav = 3;
dw_hat_3 = Ji(:,:,iiuav) * d_sigma_bar_w_vec(:,iiuav) + h3w * sigma_bar_w_hat_vec(:,iiuav);

== matlab function run_sim_paper_scenario/cal dw_hat agent 4 ==
  data: h3w input; Ji input; d_sigma_bar_w_vec input; sigma_bar_w_hat_vec input; dw_hat_4 output
function dw_hat_4 = fcn(h3w, Ji, d_sigma_bar_w_vec, sigma_bar_w_hat_vec)
%%%% rotational disturbance observation
iiuav = 4;
dw_hat_4 = Ji(:,:,iiuav) * d_sigma_bar_w_vec(:,iiuav) + h3w * sigma_bar_w_hat_vec(:,iiuav);

== matlab function run_sim_paper_scenario/cal dw_hat agent 5 ==
  data: h3w input; Ji input; d_sigma_bar_w_vec input; sigma_bar_w_hat_vec input; dw_hat_5 output
function dw_hat_5 = fcn(h3w, Ji, d_sigma_bar_w_vec, sigma_bar_w_hat_vec)
%%%% rotational disturbance observation
iiuav = 5;
dw_hat_5 = Ji(:,:,iiuav) * d_sigma_bar_w_vec(:,iiuav) + h3w * sigma_bar_w_hat_vec(:,iiuav);

== matlab function run_sim_paper_scenario/cal error dw_tilt ==
  data: dw_vec input; dw_hat_vec input; dw_tilt_vec output
function dw_tilt_vec = fcn(dw_vec, dw_hat_vec)
%%%% rotational disturbance observation error
dw_tilt_vec = zeros(3,5);
for iiuav = 1:5
    dw_tilt_vec(:,iiuav) = dw_vec(:,iiuav) - dw_hat_vec(:,iiuav);
end

== matlab function run_sim_paper_scenario/cal sig ==
  data: x input; z output; y input
function z = fcn(x, y)
z = x(:) .* sign(y(:));

== matlab function run_sim_paper_scenario/cal sig1 ==
  data: x input; z output; y input
function z = fcn(x, y)
z = x(:) .* sign(y(:));

== matlab function run_sim_paper_scenario/follower tracking error agent 3 ==
  data: ksi_track_err_3 output; delta_ksi_vec input; delta_eta_vec input; ksi_i_vec input; eta_i_vec input; ksi0 input; eta_track_err_3 output; eta0 input
function [ksi_track_err_3, eta_track_err_3]  = fcn(delta_ksi_vec, delta_eta_vec, ksi_i_vec, eta_i_vec, ksi0, eta0)
%%%% translational state tracking error for followers
eta_track_err_3 = eta_i_vec(:,3) - delta_eta_vec(:,3) - eta0;
ksi_track_err_3 = ksi_i_vec(:,3) - delta_ksi_vec(:,3) - ksi0;

== matlab function run_sim_paper_scenario/cal sig10 ==
  data: x input; z output; y input
function z = fcn(x, y)
z = x(:) .* sign(y(:));

== matlab function run_sim_paper_scenario/cal sig11 ==
  data: x input; z output; y input
function z = fcn(x, y)
z = x(:) .* sign(y(:));

== matlab function run_sim_paper_scenario/cal sig12 ==
  data: x input; z output; y input
function z = fcn(x, y)
z = x(:) .* sign(y(:));

== matlab function run_sim_paper_scenario/cal sig13 ==
  data: x input; z output; y input
function z = fcn(x, y)
z = x(:) .* sign(y(:));

== matlab function run_sim_paper_scenario/cal sig14 ==
  data: x input; z output; y input
function z = fcn(x, y)
z = x(:) .* sign(y(:));

== matlab function run_sim_paper_scenario/cal sig15 ==
  data: x input; z output; y input
function z = fcn(x, y)
z = x(:) .* sign(y(:));

== matlab function run_sim_paper_scenario/cal sig16 ==
  data: x input; z output; y input
function z = fcn(x, y)
z = x(:) .* sign(y(:));

== matlab function run_sim_paper_scenario/cal sig17 ==
  data: x input; z output; y input
function z = fcn(x, y)
z = x(:) .* sign(y(:));

== matlab function run_sim_paper_scenario/cal sig18 ==
  data: x input; z output; y input
function z = fcn(x, y)
z = x(:) .* sign(y(:));

== matlab function run_sim_paper_scenario/cal sig19 ==
  data: x input; z output; y input
function z = fcn(x, y)
z = x(:) .* sign(y(:));

== matlab function run_sim_paper_scenario/cal sig2 ==
  data: x input; z output; y input
function z = fcn(x, y)
z = x(:) .* sign(y(:));

== matlab function run_sim_paper_scenario/cal sig20 ==
  data: x input; z output; y input
function z = fcn(x, y)
z = x(:) .* sign(y(:));

== matlab function run_sim_paper_scenario/cal sig21 ==
  data: x input; z output; y input
function z = fcn(x, y)
z = x(:) .* sign(y(:));

== matlab function run_sim_paper_scenario/cal sig22 ==
  data: x input; z output; y input
function z = fcn(x, y)
z = x(:) .* sign(y(:));

== matlab function run_sim_paper_scenario/cal sig23 ==
  data: x input; z output; y input
function z = fcn(x, y)
z = x(:) .* sign(y(:));

== matlab function run_sim_paper_scenario/cal sig24 ==
  data: x input; z output; y input
function z = fcn(x, y)
z = x(:) .* sign(y(:));

== matlab function run_sim_paper_scenario/follower tracking error agent 4 ==
  data: ksi_track_err_4 output; delta_ksi_vec input; delta_eta_vec input; ksi_i_vec input; eta_i_vec input; ksi0 input; eta_track_err_4 output; eta0 input
function [ksi_track_err_4, eta_track_err_4]  = fcn(delta_ksi_vec, delta_eta_vec, ksi_i_vec, eta_i_vec, ksi0, eta0)
%%%% translational state tracking error for followers
eta_track_err_4 = eta_i_vec(:,4) - delta_eta_vec(:,4) - eta0;
ksi_track_err_4 = ksi_i_vec(:,4) - delta_ksi_vec(:,4) - ksi0;

== matlab function run_sim_paper_scenario/cal sig25 ==
  data: x input; z output; y input
function z = fcn(x, y)
z = x(:) .* sign(y(:));

== matlab function run_sim_paper_scenario/cal sig26 ==
  data: x input; z output; y input
function z = fcn(x, y)
z = x(:) .* sign(y(:));

== matlab function run_sim_paper_scenario/cal sig27 ==
  data: x input; z output; y input
function z = fcn(x, y)
z = x(:) .* sign(y(:));

== matlab function run_sim_paper_scenario/cal sig28 ==
  data: x input; z output; y input
function z = fcn(x, y)
z = x(:) .* sign(y(:));

== matlab function run_sim_paper_scenario/cal sig29 ==
  data: x input; z output; y input
function z = fcn(x, y)
z = x(:) .* sign(y(:));

== matlab function run_sim_paper_scenario/cal sig3 ==
  data: x input; z output; y input
function z = fcn(x, y)
z = x(:) .* sign(y(:));

== matlab function run_sim_paper_scenario/cal sig4 ==
  data: x input; z output; y input
function z = fcn(x, y)
z = x(:) .* sign(y(:));

== matlab function run_sim_paper_scenario/cal sig5 ==
  data: x input; z output; y input
function z = fcn(x, y)
z = x(:) .* sign(y(:));

== matlab function run_sim_paper_scenario/cal sig6 ==
  data: x input; z output; y input
function z = fcn(x, y)
z = x(:) .* sign(y(:));

== matlab function run_sim_paper_scenario/cal sig7 ==
  data: x input; z output; y input
function z = fcn(x, y)
z = x(:) .* sign(y(:));

== matlab function run_sim_paper_scenario/cal sig8 ==
  data: x input; z output; y input
function z = fcn(x, y)
z = x(:) .* sign(y(:));

== matlab function run_sim_paper_scenario/cal sig9 ==
  data: x input; z output; y input
function z = fcn(x, y)
z = x(:) .* sign(y(:));

== matlab function run_sim_paper_scenario/cal sigma_bar_w_hat agent 1 ==
  data: h1w input; h2w input; theta_sigma_bar_w_tilt_1_vec input; d_sigma_bar_w_hat_1 output; theta_sigma_bar_w_tilt_2_vec input; d_sigma_bar_w_vec input
function d_sigma_bar_w_hat_1 = fcn(h1w, h2w, theta_sigma_bar_w_tilt_1_vec, theta_sigma_bar_w_tilt_2_vec, d_sigma_bar_w_vec)
%%%% observation of virtual angular velocity control variable
iiuav = 1;
d_sigma_bar_w_hat_1 = d_sigma_bar_w_vec(:,iiuav) + ...
                                            h1w * theta_sigma_bar_w_tilt_1_vec(:,iiuav) + ...
                                            h2w * theta_sigma_bar_w_tilt_2_vec(:,iiuav);

== matlab function run_sim_paper_scenario/cal sigma_bar_w_hat agent 2 ==
  data: h1w input; h2w input; theta_sigma_bar_w_tilt_1_vec input; d_sigma_bar_w_hat_2 output; theta_sigma_bar_w_tilt_2_vec input; d_sigma_bar_w_vec input
function d_sigma_bar_w_hat_2 = fcn(h1w, h2w, theta_sigma_bar_w_tilt_1_vec, theta_sigma_bar_w_tilt_2_vec, d_sigma_bar_w_vec)
%%%% observation of virtual angular velocity control variable
iiuav = 2;
d_sigma_bar_w_hat_2 = d_sigma_bar_w_vec(:,iiuav) + ...
                                            h1w * theta_sigma_bar_w_tilt_1_vec(:,iiuav) + ...
                                            h2w * theta_sigma_bar_w_tilt_2_vec(:,iiuav);

== matlab function run_sim_paper_scenario/cal sigma_bar_w_hat agent 3 ==
  data: h1w input; h2w input; theta_sigma_bar_w_tilt_1_vec input; d_sigma_bar_w_hat_3 output; theta_sigma_bar_w_tilt_2_vec input; d_sigma_bar_w_vec input
function d_sigma_bar_w_hat_3 = fcn(h1w, h2w, theta_sigma_bar_w_tilt_1_vec, theta_sigma_bar_w_tilt_2_vec, d_sigma_bar_w_vec)
%%%% observation of virtual angular velocity control variable
iiuav = 3;
d_sigma_bar_w_hat_3 = d_sigma_bar_w_vec(:,iiuav) + ...
                                            h1w * theta_sigma_bar_w_tilt_1_vec(:,iiuav) + ...
                                            h2w * theta_sigma_bar_w_tilt_2_vec(:,iiuav);

== matlab function run_sim_paper_scenario/follower tracking error agent 5 ==
  data: ksi_track_err_5 output; delta_ksi_vec input; delta_eta_vec input; ksi_i_vec input; eta_i_vec input; ksi0 input; eta_track_err_5 output; eta0 input
function [ksi_track_err_5, eta_track_err_5]  = fcn(delta_ksi_vec, delta_eta_vec, ksi_i_vec, eta_i_vec, ksi0, eta0)
%%%% translational state tracking error for followers
eta_track_err_5 = eta_i_vec(:,5) - delta_eta_vec(:,5) - eta0;
ksi_track_err_5 = ksi_i_vec(:,5) - delta_ksi_vec(:,5) - ksi0;

== matlab function run_sim_paper_scenario/cal sigma_bar_w_hat agent 4 ==
  data: h1w input; h2w input; theta_sigma_bar_w_tilt_1_vec input; d_sigma_bar_w_hat_4 output; theta_sigma_bar_w_tilt_2_vec input; d_sigma_bar_w_vec input
function d_sigma_bar_w_hat_4 = fcn(h1w, h2w, theta_sigma_bar_w_tilt_1_vec, theta_sigma_bar_w_tilt_2_vec, d_sigma_bar_w_vec)
%%%% observation of virtual angular velocity control variable
iiuav = 4;
d_sigma_bar_w_hat_4 = d_sigma_bar_w_vec(:,iiuav) + ...
                                            h1w * theta_sigma_bar_w_tilt_1_vec(:,iiuav) + ...
                                            h2w * theta_sigma_bar_w_tilt_2_vec(:,iiuav);

== matlab function run_sim_paper_scenario/cal sigma_bar_w_hat agent 5 ==
  data: h1w input; h2w input; theta_sigma_bar_w_tilt_1_vec input; d_sigma_bar_w_hat_5 output; theta_sigma_bar_w_tilt_2_vec input; d_sigma_bar_w_vec input
function d_sigma_bar_w_hat_5 = fcn(h1w, h2w, theta_sigma_bar_w_tilt_1_vec, theta_sigma_bar_w_tilt_2_vec, d_sigma_bar_w_vec)
%%%% observation of virtual angular velocity control variable
iiuav = 5;
d_sigma_bar_w_hat_5 = d_sigma_bar_w_vec(:,iiuav) + ...
                                            h1w * theta_sigma_bar_w_tilt_1_vec(:,iiuav) + ...
                                            h2w * theta_sigma_bar_w_tilt_2_vec(:,iiuav);

== matlab function run_sim_paper_scenario/cal sigma_w_bar ==
  data: sigma_bar_w_vec output; wi_vec input; sigma_w_vec input
function sigma_bar_w_vec = fcn(wi_vec, sigma_w_vec)
%%%% tracking error : auxiliary angular velocity tracking real velocity
sigma_bar_w_vec = zeros(3,5);
for iiuav = 1:5
    sigma_bar_w_vec(:,iiuav) = wi_vec(:,iiuav) - sigma_w_vec(:,iiuav);
end
